simulink model "HW10_488"  (R2024a)
settings: Solver=VariableStepAuto  StartTime=0.0  StopTime=stop_time  MaxStep=max_step_size  RelTol=1e-3
values from neighbouring files (symbols this model uses):
  I = 6e-5    (= 6e-05)    [MAE488_Nicholas_Hawse_HW10.m]    (also in MAE488_Nicholas_Hawse_HW5.m = 8e-05)
  InputCommand = 1    [MAE488_Nicholas_Hawse_HW10.m]
  K1 = 0.0576    [MAE488_Nicholas_Hawse_HW10.m]
  K2 = 0.00516    [MAE488_Nicholas_Hawse_HW10.m]
  K3 = -0.476    [MAE488_Nicholas_Hawse_HW10.m]
  K_I = 0.096    [MAE488_Nicholas_Hawse_HW10.m]
  K_T = 0.04    [MAE488_Nicholas_Hawse_HW10.m]
  L = 2e-3    (= 0.002)    [MAE488_Nicholas_Hawse_HW10.m]
  R = 0.6    [MAE488_Nicholas_Hawse_HW10.m]
  satLower = -2    [MAE488_Nicholas_Hawse_HW10.m]
  satUpper = 2    [MAE488_Nicholas_Hawse_HW10.m]
  T_d = 0.1    [MAE488_Nicholas_Hawse_HW10.m]
settings Model: Creator=nicholas  LastModifiedBy=nicholas

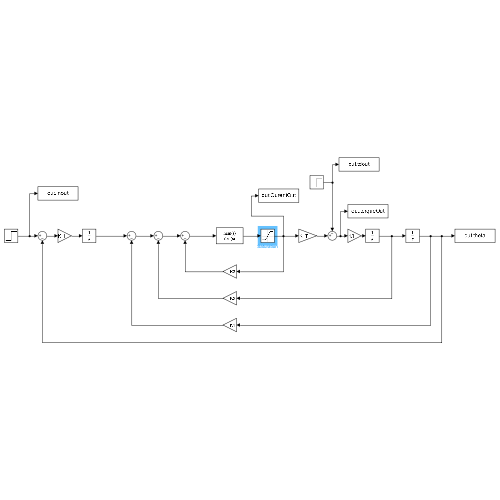
[thumbnail: Simulink's stored preview of the top-level diagram]
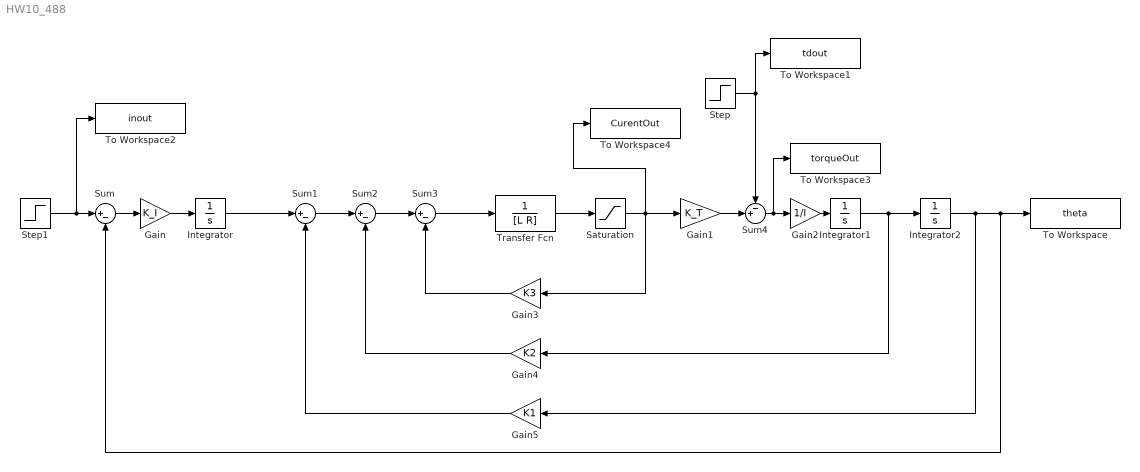
== system HW10_488 ==
  Gain : Gain  Gain=K_I
  Gain1 : Gain  Gain=K_T
  Gain2 : Gain  Gain=1/I
  Gain3 : Gain  Gain=K3
  Gain4 : Gain  Gain=K2
  Gain5 : Gain  Gain=K1
  Integrator : Integrator
  Integrator1 : Integrator
  Integrator2 : Integrator
  Saturation : Saturate  UpperLimit=satUpper  LowerLimit=satLower
  Step : Step  Time=0  After=T_d  SampleTime=0
  Step1 : Step  Time=0  After=InputCommand  SampleTime=0
  Sum{,1..3} (4 alike) : Sum  Inputs=|+-
  Sum4 : Sum  Inputs=-+|
  To Workspace : ToWorkspace  VariableName=theta  SaveFormat=Timeseries  SampleTime=-1
  To Workspace1 : ToWorkspace  VariableName=tdout  SaveFormat=Timeseries  SampleTime=-1
  To Workspace2 : ToWorkspace  VariableName=inout  SaveFormat=Timeseries  SampleTime=-1
  To Workspace3 : ToWorkspace  VariableName=torqueOut  SaveFormat=Timeseries  SampleTime=-1
  To Workspace4 : ToWorkspace  VariableName=CurentOut  SaveFormat=Timeseries  SampleTime=-1
  Transfer Fcn : TransferFcn  Denominator=[L R]
  wires:
  Sum/1 -> Gain/1
  Gain/1 -> Integrator/1
  Integrator/1 -> Sum1/1
  Sum1/1 -> Sum2/1
  Sum2/1 -> Sum3/1
  Sum3/1 -> Transfer Fcn/1
  Transfer Fcn/1 -> Saturation/1
  Saturation/1 -> To Workspace4/1, Gain3/1, Gain1/1
  Gain1/1 -> Sum4/2
  Sum4/1 -> To Workspace3/1, Gain2/1
  Gain2/1 -> Integrator1/1
  Integrator1/1 -> Gain4/1, Integrator2/1
  Gain3/1 -> Sum3/2
  Gain4/1 -> Sum2/2
  Gain5/1 -> Sum1/2
  Integrator2/1 -> Gain5/1, To Workspace/1, Sum/2
  Step/1 -> Sum4/1, To Workspace1/1
  Step1/1 -> To Workspace2/1, Sum/1
